simulink model "dB_lookup_table"  (R2020b)
settings: Solver=FixedStepAuto  StartTime=0.0  StopTime=stop_time  RelTol=1e-3
InitFcn:
  | test_FFT_to_gain_init
StopFcn:
  | test_FFT_to_gain_stop
undefined symbols (not defined in the file or in its folder): xIn
libraries: FPGA_Open_Speech_Tools x1
settings Model: Creator=t96f346  LastModifiedBy=wickh
settings DataIOCC: SaveOutput=off  SaveTime=off

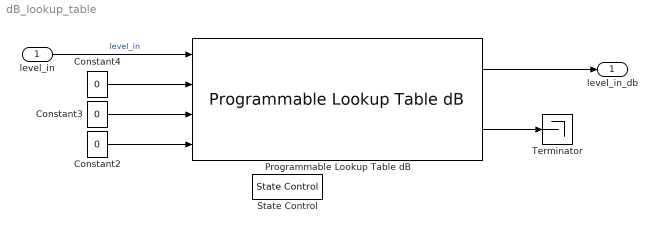
== system dB_lookup_table ==
  level_in : Inport  OutDataTypeStr=fixdt(1,40,32)  PortDimensions=1
  Constant2 : Constant  Value=0  OutDataTypeStr=boolean  SampleTime=-1
  Constant3 : Constant  Value=0  OutDataTypeStr=uint16  SampleTime=-1
  Constant4 : Constant  Value=0  OutDataTypeStr=fixdt(1,40,32)  SampleTime=-1
  Programmable Lookup Table dB : FPGA_Open_Speech_Tools/Programmable Lookup Table dB  tableFnParam=10.*log10(2500000000.*xIn)  SAVE_TABLE=off  maxInput=1  floorParam=2^-31  errorParam=1  ERR_DIAG=on  PLOT_TABLE=off  nBitsParam=5  mBitsParam=4  IGOTTHIS=off  W_bits=40  F_bits=37  tableInit=0  binaryOffset=0
      link override High_LUT/ram_data: InitialCondition=55.36
      link override Linear_Approximation/Unit Delay: InitialCondition=65
      link override LogAddressing/Delay1: InitialCondition=13
      link override LogAddressing/Delay2: InitialCondition=0.0001265
      link override Low_LUT/ram_data: InitialCondition=54.85
      link override Unit Delay1: InitialCondition=0.0001265
      link override Unit Delay2: InitialCondition=0.0001265
      link override Unit Delay3: InitialCondition=144
      settings: SourceProductName=FPGA Open Speech Tools
  State Control : StateControl  StateControl=Synchronous
  Terminator : Terminator
  level_in_db : Outport  OutDataTypeStr=fixdt(1,40,32)  PortDimensions=1
  wires:
  Constant2/1 -> Programmable Lookup Table dB/4
  Constant3/1 -> Programmable Lookup Table dB/3
  Constant4/1 -> Programmable Lookup Table dB/2
  Programmable Lookup Table dB/1 -> level_in_db/1
  level_in/1 -> Programmable Lookup Table dB/1  "level_in"
  Programmable Lookup Table dB/2 -> Terminator/1
